simulink model "Function3"  (R2020b)
settings: Solver=FixedStepDiscrete  StartTime=0.0  StopTime=0.1  FixedStep=0.1  RelTol=1e-3  EnableMultiTasking=on
settings Model: Creator=bzhan  LastModifiedBy=apple
settings SolverCC: AutoInsertRateTranBlk=on
settings DataIOCC: LimitDataPoints=on
settings OptimizationCC: LifeSpan=inf
settings DebuggingCC: AllowSymbolicDim=off  SFUnexpectedBacktrackingDiag=warning  SFNoUnconditionalDefaultTransitionDiag=warning  SFExecutionAtInitializationDiag=none  ArithmeticOperatorsInVariantConditions=warning
settings SFSimCC: SimUseLocalCustomCode=off  CustomCodeUndefinedFunction=UseInterfaceOnly
settings RTWCC: RTWUseLocalCustomCode=off
settings CodeAppCC: StateflowObjectComments=on
settings GRTTargetCC: TargetLangStandard=C89/C90 (ANSI)
settings ConfigComp: CovMetricSettings=dw  CovSaveCumulativeToWorkspaceVar=on  CovSaveSingleToWorkspaceVar=on  CovExternalEMLEnable=off  CovSFcnEnable=off

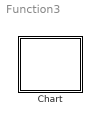
== system Function3 ==
  Chart : Stateflow chart  TreatAsAtomicUnit=on

== stateflow chart Function3/Chart ==
  state A
    en: f("en_A")
  state B
    en: f("en_B")
  (default) -> A
  (junction 29) -> B : [a1==0 && a2==2 && a3 == 4]
  A -> (junction 29) : {compute()}
  data: s function_input; a1 local; a3 local; a2 local
  function compute:
    | function compute
    |   a1 = 0;
    |   a2 = 1+1;
    |   a3 = 2+2;
  function f(s):
    | function f(s)
    |   fprintf(s+"\n");
